simulink model "AutoPID_FOC_Model_Voltage"  (R2022b)
settings: Solver=ode15s  StartTime=0.0  StopTime=5  MaxStep=1e-5  RelTol=1e-4
undefined symbols (not defined in the file): J, kc, p, PID_angle_limit, PID_vel_D, PID_vel_I, PID_vel_limit, PID_vel_output_ramp, PID_vel_P, step_final, Ts_control
libraries: fl_lib x6, nesl_utility x6, slpidlib x2, mcbcontrolslib x2, ee_lib x1
settings Model: Creator=ngryaznov  LastModifiedBy=ngryaznov
settings DataIOCC: SaveOutput=off  SignalLogging=off  SaveTime=off

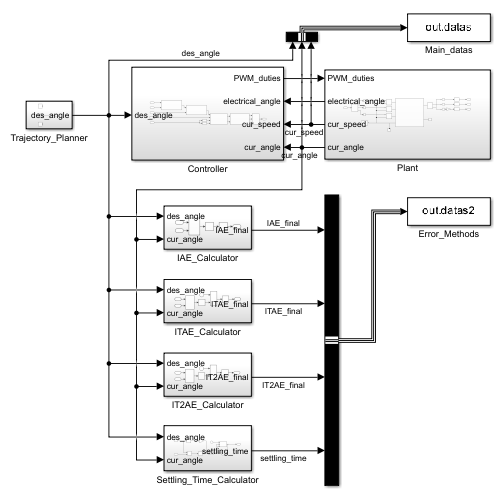
[thumbnail: Simulink's stored preview of the top-level diagram]
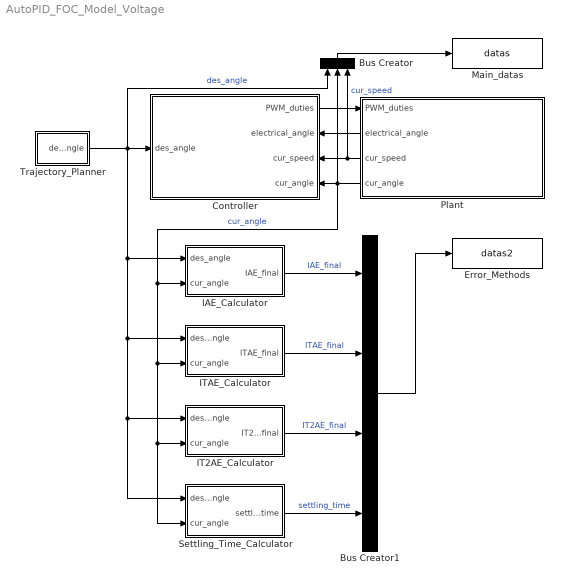
== system AutoPID_FOC_Model_Voltage ==
  Bus Creator : BusCreator  Inputs=3
  Bus Creator1 : BusCreator  Inputs=4
  Controller : Subsystem
      settings: PortSchema="{\"entries\":[{\"content\":{\"sides\":[{\"content\":{\"connectorIds\":[\"In1\"]},\"type\":\"ConnectorPlacement.EquallySpacedRectSide\",\"uuid\":\"0423d24d-9521-4525-a0e4-a3e2e668f0ac\"},{\"content\":{\"connectorIds\":[\"Out1\",\"In2\",\"In3\",\"In4\"],\"side\":\"RIGHT\"},\"type\":\"ConnectorPlacement.EquallySpacedRectSide\",\"uuid\":\"47c71c52-a907-4714-8b3c-a2837c55c5aa\"},{\"content\":{\"connectorIds\":[],\"side\":\"TOP\"},\"type\":\"ConnectorPlacement.EquallySpacedRectSide\",\"uuid\":\"3c8a956e-8d48-45c8-90f9-0152c5abea5b\"}]},\"type\":\"ConnectorPlacement.EquallySpacedConnector\",\"uuid\":\"215a3bc6-e4d0-4bbf-a22d-a4a170c152a2\"}],\"packageUris\":[\"http://schema.mathworks.com/mf0/Connector/R2020b\"],\"version\":\"1.0\"}"
  Error_Methods : ToWorkspace  VariableName=datas2  SaveFormat=Timeseries  SampleTime=-1
      settings: Decimation=2
  IAE_Calculator : Subsystem
  IT2AE_Calculator : Subsystem
  ITAE_Calculator : Subsystem
  Main_datas : ToWorkspace  VariableName=datas  SaveFormat=Timeseries  SampleTime=-1
      settings: Decimation=2
  Plant : Subsystem
      settings: PortSchema="{\"entries\":[{\"content\":{\"sides\":[{\"content\":{\"connectorIds\":[\"In1\",\"Out1\",\"Out2\",\"Out3\"]},\"type\":\"ConnectorPlacement.EquallySpacedRectSide\",\"uuid\":\"e046dd69-40e9-406a-bd4f-9d09bb11ef1b\"},{\"content\":{\"connectorIds\":[],\"side\":\"RIGHT\"},\"type\":\"ConnectorPlacement.EquallySpacedRectSide\",\"uuid\":\"7e51beb7-44f5-4f8e-b575-c3917b5b8c79\"},{\"content\":{\"connectorIds\":[],\"side\":\"TOP\"},\"type\":\"ConnectorPlacement.EquallySpacedRectSide\",\"uuid\":\"ce36b3ae-82b4-4f86-a013-a2335df0f3e3\"}]},\"type\":\"ConnectorPlacement.EquallySpacedConnector\",\"uuid\":\"95338947-5a02-4018-9bff-e920c50d3b4f\"}],\"packageUris\":[\"http://schema.mathworks.com/mf0/Connector/R2020b\"],\"version\":\"1.0\"}"
  Settling_Time_Calculator : Subsystem
  Trajectory_Planner : Subsystem
  wires:
  Trajectory_Planner/1(des_angle) -> ITAE_Calculator/1(des_angle), IT2AE_Calculator/1(des_angle), Settling_Time_Calculator/1(des_angle), IAE_Calculator/1(des_angle), Controller/1(des_angle), Bus Creator/1  "des_angle"
  Controller/1(PWM_duties) -> Plant/1(PWM_duties)
  Plant/1(electrical_angle) -> Controller/2(electrical_angle)
  Plant/2(cur_speed) -> Bus Creator/3, Controller/3(cur_speed)  "cur_speed"
  Plant/3(cur_angle) -> Bus Creator/2, Controller/4(cur_angle), IAE_Calculator/2(cur_angle), ITAE_Calculator/2(cur_angle), IT2AE_Calculator/2(cur_angle), Settling_Time_Calculator/2(cur_angle)  "cur_angle"
  Bus Creator/1 -> Main_datas/1
  IAE_Calculator/1(IAE_final) -> Bus Creator1/1  "IAE_final"
  ITAE_Calculator/1(ITAE_final) -> Bus Creator1/2  "ITAE_final"
  IT2AE_Calculator/1(IT2AE_final) -> Bus Creator1/3  "IT2AE_final"
  Settling_Time_Calculator/1(settling_time) -> Bus Creator1/4  "settling_time"
  Bus Creator1/1 -> Error_Methods/1

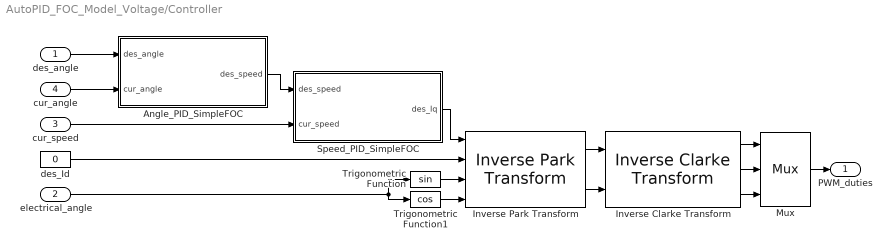
== system AutoPID_FOC_Model_Voltage/Controller ==
  des_angle : Inport
  electrical_angle : Inport  Port=2
  cur_speed : Inport  Port=3
  cur_angle : Inport  Port=4
  Angle_PID_SimpleFOC : Subsystem
  Inverse Clarke Transform : mcbcontrolslib/Inverse Clarke Transform
      settings: LibrarySourceBlock=mcblib/Controls/Math Transforms/Inverse Clarke Transform
  Inverse Park Transform : mcbcontrolslib/Inverse Park Transform  AxisAlignment=Q-axis
      settings: LibrarySourceBlock=mcblib/Controls/Math Transforms/Inverse Park Transform
  Mux : Mux  Inputs=3
      settings: DisplayOption=signals
  Speed_PID_SimpleFOC : Subsystem
  Trigonometric Function : Trigonometry
  Trigonometric Function1 : Trigonometry  Operator=cos
  des_Id : Constant  Value=0
  PWM_duties : Outport
  wires:
  des_angle/1 -> Angle_PID_SimpleFOC/1(des_angle)
  cur_angle/1 -> Angle_PID_SimpleFOC/2(cur_angle)
  des_Id/1 -> Inverse Park Transform/2
  electrical_angle/1 -> Trigonometric Function1/1, Trigonometric Function/1
  Trigonometric Function/1 -> Inverse Park Transform/3
  Trigonometric Function1/1 -> Inverse Park Transform/4
  Inverse Park Transform/2 -> Inverse Clarke Transform/2
  Mux/1 -> PWM_duties/1
  Inverse Clarke Transform/1 -> Mux/1
  Inverse Clarke Transform/3 -> Mux/3
  Inverse Clarke Transform/2 -> Mux/2
  Angle_PID_SimpleFOC/1(des_speed) -> Speed_PID_SimpleFOC/1(des_speed)
  cur_speed/1 -> Speed_PID_SimpleFOC/2(cur_speed)
  Inverse Park Transform/1 -> Inverse Clarke Transform/1
  Speed_PID_SimpleFOC/1(des_Iq) -> Inverse Park Transform/1

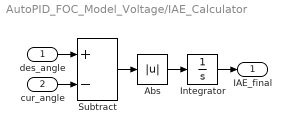
== system AutoPID_FOC_Model_Voltage/IAE_Calculator ==
  des_angle : Inport
  cur_angle : Inport  Port=2
  Abs : Abs  SaturateOnIntegerOverflow=off
  Integrator : Integrator
  Subtract : Sum  Inputs=+-
  IAE_final : Outport
  wires:
  Subtract/1 -> Abs/1
  des_angle/1 -> Subtract/1
  cur_angle/1 -> Subtract/2
  Integrator/1 -> IAE_final/1
  Abs/1 -> Integrator/1

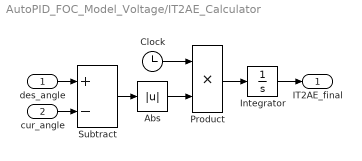
== system AutoPID_FOC_Model_Voltage/IT2AE_Calculator ==
  des_angle : Inport
  cur_angle : Inport  Port=2
  Abs : Abs  SaturateOnIntegerOverflow=off
  Clock : Clock
  Integrator : Integrator
  Product : Product
  Subtract : Sum  Inputs=+-
  IT2AE_final : Outport
  wires:
  des_angle/1 -> Subtract/1
  cur_angle/1 -> Subtract/2
  Subtract/1 -> Abs/1
  Abs/1 -> Product/2
  Clock/1 -> Product/1
  Integrator/1 -> IT2AE_final/1
  Product/1 -> Integrator/1

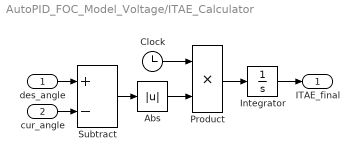
== system AutoPID_FOC_Model_Voltage/ITAE_Calculator ==
  des_angle : Inport
  cur_angle : Inport  Port=2
  Abs : Abs  SaturateOnIntegerOverflow=off
  Clock : Clock
  Integrator : Integrator
  Product : Product
  Subtract : Sum  Inputs=+-
  ITAE_final : Outport
  wires:
  Integrator/1 -> ITAE_final/1
  cur_angle/1 -> Subtract/2
  Subtract/1 -> Abs/1
  des_angle/1 -> Subtract/1
  Abs/1 -> Product/2
  Product/1 -> Integrator/1
  Clock/1 -> Product/1

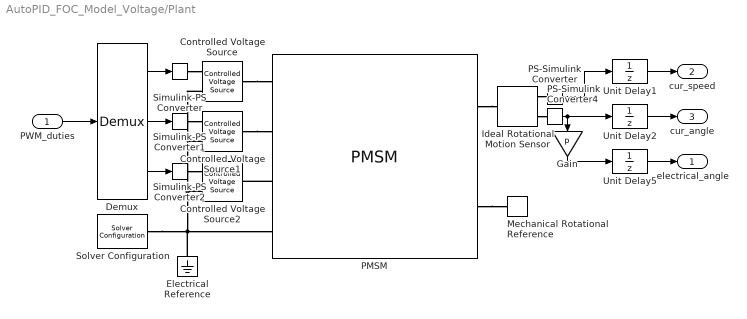
== system AutoPID_FOC_Model_Voltage/Plant ==
  PWM_duties : Inport
  Controlled Voltage Source : fl_lib/Electrical/Electrical Sources/Controlled Voltage Source
  Controlled Voltage Source1 : fl_lib/Electrical/Electrical Sources/Controlled Voltage Source
  Controlled Voltage Source2 : fl_lib/Electrical/Electrical Sources/Controlled Voltage Source
  Demux : Demux  Outputs=3
      settings: DisplayOption=none
  Electrical Reference : fl_lib/Electrical/Electrical Elements/Electrical Reference
  Gain : Gain  Gain=p
  Ideal Rotational Motion Sensor : fl_lib/Mechanical/Mechanical Sensors/Ideal Rotational Motion Sensor  reference=foundation.enum.MeasurementReference.absolute  acceleration_port=false  velocity_port=true  position_port=true  wrap_angle=false  offset=0 rad
      settings: InternalSimscapePortConfiguration="{\"Bottom\":[],\"Left\":[{\"id\":\"R\",\"label\":\"R\",\"type\":\"foundation.mechanical.rotational.rotational\"}],\"Right\":[{\"id\":\"W\",\"label\":\"W\",\"type\":\"output\"},{\"id\":\"A\",\"label\":\"A\",\"type\":\"output\"}],\"Top\":[]}"
  Mechanical Rotational Reference : fl_lib/Mechanical/Rotational Elements/Mechanical Rotational Reference
  PMSM : ee_lib/Electromechanical/Permanent Magnet/PMSM  port_option=ee.enum.threePhasePort.expanded  winding_type=ee.enum.statorconnection.wye  machine_param=ee.enum.pmsm.parameterization.constant  nPolePairs=p  pmflux_param=ee.enum.pmflux.fluxlinkage  pm_flux_linkage=lambda_pm Wb  torque_constant=0.18 N*m/A  back_emf_constant=0.18 V*s/rad  stator_param=ee.enum.statorparam.LdLqL0  Ld=Ld H  Lq=Lq H  idVec=[-200, 0, 200] A  iqVec=[-200, 0, 200] A  LdMatrix=0.0002 * ones(3, 3) H  LqMatrix=0.0002 * ones(3, 3) H  PmMatrix=0.1 * ones(3, 3) Wb  ktMatrix=0.18 * ones(3, 3) N*m/A  keMatrix=0.18 * ones(3, 3) V*s/rad  L0=Ld H  Ls=0.0002 H  Lm=-0.00002 H  Ms=0.00002 H  Rs=Rs Ohm  zero_sequence=ee.enum.park.zerosequence.include  axes_param=ee.enum.rotorangle.daxis  loss_param=ee.enum.ironloss.none  losses_oc=[0, 0, 0] W  losses_sc=[0, 0, 0] W  f_losses=60 Hz  Isc_losses=95 A  J=J kg*m^2  lam=B N*m*s/rad  i_d_specify=off  i_d_priority=None  i_d=0 A  i_d_nominal_specify=off  i_d_nominal_unit=A  i_d_nominal_value=1  i_q_specify=off  i_q_priority=None  i_q=0 A  i_q_nominal_specify=off  i_q_nominal_unit=A  i_q_nominal_value=1  torque_specify=off  torque_priority=None  torque=0 N*m  torque_nominal_specify=off  torque_nominal_unit=N*m  torque_nominal_value=1  angular_velocity_specify=off  angular_velocity_priority=High  angular_velocity=0 rpm  angular_velocity_nominal_specify=off  angular_velocity_nominal_unit=rpm  angular_velocity_nominal_value=1  angular_position_specify=off  angular_position_priority=High  angular_position=0 deg  angular_position_nominal_specify=off  angular_position_nominal_unit=deg  angular_position_nominal_value=1  alpha=3.93e-3 1/K  alpha_flux=-0.001 1/K  Tmeas=298.15 K  stator_thermal_mass=100 J/K  rotor_thermal_mass=200 J/K  Rm_percent_rotor=90  Rd_percent_rotor=30  temperatureA_specify=off  temperatureA_priority=High  temperatureA=25 degC  temperatureA_nominal_specify=off  temperatureA_nominal_unit=degC  temperatureA_nominal_value=1  temperatureB_specify=off  temperatureB_priority=High  temperatureB=25 degC  temperatureB_nominal_specify=off  temperatureB_nominal_unit=degC  temperatureB_nominal_value=1  temperatureC_specify=off  temperatureC_priority=High  temperatureC=25 degC  temperatureC_nominal_specify=off  temperatureC_nominal_unit=degC  temperatureC_nominal_value=1  temperatureR_specify=off  temperatureR_priority=High  temperatureR=25 degC  temperatureR_nominal_specify=off  temperatureR_nominal_unit=degC  temperatureR_nominal_value=1
      settings: InternalSimscapePortConfiguration="{\"Bottom\":[],\"Left\":[{\"id\":\"a\",\"label\":\"a\",\"type\":\"foundation.electrical.electrical\"},{\"id\":\"b\",\"label\":\"b\",\"type\":\"foundation.electrical.electrical\"},{\"id\":\"c\",\"label\":\"c\",\"type\":\"foundation.electrical.electrical\"},{\"id\":\"n\",\"label\":\"n\",\"type\":\"foundation.electrical.electrical\"}],\"Right\":[{\"id\":\"R\",\"label\":\"R\",\"type\":\"foundation.mechanical.rotational.rotational\"},{\"id\":\"C\",\"label\":\"C\",\"type\":\"foundation.mechanical.rotational.rotational\"}],\"Top\":[]}"
  PS-Simulink Converter : nesl_utility/PS-Simulink Converter  PhysicalDomain=network_engine_domain  SubClassName=ps_output  LeftPortType=input  RightPortType=output  PseudoPeriodic=off  Frequencies=[]  VectorFormat=inherit  Unit=inherit  AffineConversion=off
  PS-Simulink Converter4 : nesl_utility/PS-Simulink Converter  PhysicalDomain=network_engine_domain  SubClassName=ps_output  LeftPortType=input  RightPortType=output  PseudoPeriodic=off  Frequencies=[]  VectorFormat=inherit  Unit=inherit  AffineConversion=off
  Simulink-PS Converter : nesl_utility/Simulink-PS Converter  PhysicalDomain=network_engine_domain  SubClassName=ps_input  LeftPortType=input  RightPortType=output  PseudoPeriodic=off  Frequencies=[]  NoiseDistribution=none  NoiseParameters=[]  Unit=1  AffineConversion=off  FilteringAndDerivatives=provide  SimscapeFilterOrder=1  InputFilterTimeConstant=0.001  UdotUserProvided=0
  Simulink-PS Converter1 : nesl_utility/Simulink-PS Converter  PhysicalDomain=network_engine_domain  SubClassName=ps_input  LeftPortType=input  RightPortType=output  PseudoPeriodic=off  Frequencies=[]  NoiseDistribution=none  NoiseParameters=[]  Unit=1  AffineConversion=off  FilteringAndDerivatives=provide  SimscapeFilterOrder=1  InputFilterTimeConstant=0.001  UdotUserProvided=0
  Simulink-PS Converter2 : nesl_utility/Simulink-PS Converter  PhysicalDomain=network_engine_domain  SubClassName=ps_input  LeftPortType=input  RightPortType=output  PseudoPeriodic=off  Frequencies=[]  NoiseDistribution=none  NoiseParameters=[]  Unit=1  AffineConversion=off  FilteringAndDerivatives=provide  SimscapeFilterOrder=1  InputFilterTimeConstant=0.001  UdotUserProvided=0
  Solver Configuration : nesl_utility/Solver Configuration  PhysicalDomain=network_engine_domain  SubClassName=solver  LeftPortType=input  RightPortType=generic  Tones=[]  Harmonics=[]  SimulateNoise=off  Profile=off  UseLocalSampling=off  EnableSwitchedLinearOptims=on  FrequencyDomain=off  UseCCode=off  RelTol=0.001  AbsTol=0.001  MinStep=1e-09  ToWorkspace=off  RevertToSquareIcSolve=off  NumHomotopyIterations=100  PhasorMode=off  PhasorModeNumHarmonics=1  ConsistencySolver=NEWTON_XTOL_AFTER_FTOL  IndexReductionMethod=DerivativeReplacement  DoDC=off  ResidualTolerance=1e-09  ConsistencyTolSource=GLOBAL  ConsistencyAbsTol=0.001  ConsistencyRelTol=0.001  ConsistencyTolFactor=0.001  UseLocalSolver=on  LocalSolverChoice=NE_BACKWARD_EULER_ADVANCER  ResolveIndetEquations=on  FunctionEvalNumThread=1  LocalSolverSampleTime=0.001  DoFixedCost=on  MaxNonlinIter=3  MaxModeIter=2  ComputeImpulses=off  ImpulseIterations=2  LinearAlgebra=auto  LinearAlgebraNumThread=0  EquationFormulation=NE_TIME_EF  DelaysMemoryBudget=1024  AutomaticFiltering=on  FilteringTimeConstant=0.001  PartitionStorageMethod=AS_NEEDED  PartitionMemoryBudget=1024  PartitionMethod=ROBUST
  Unit Delay1 : UnitDelay  SampleTime=Ts_control  HasFrameUpgradeWarning=on
  Unit Delay2 : UnitDelay  SampleTime=Ts_control  HasFrameUpgradeWarning=on
  Unit Delay5 : UnitDelay  SampleTime=Ts_control  HasFrameUpgradeWarning=on
  electrical_angle : Outport
  cur_speed : Outport  Port=2
  cur_angle : Outport  Port=3
  wires:
  PS-Simulink Converter/1 -> Unit Delay1/1
  PS-Simulink Converter4/1 -> Unit Delay2/1, Gain/1
  PWM_duties/1 -> Demux/1
  Gain/1 -> Unit Delay5/1
  Demux/1 -> Simulink-PS Converter/1
  Demux/2 -> Simulink-PS Converter1/1
  Demux/3 -> Simulink-PS Converter2/1
  Unit Delay1/1 -> cur_speed/1
  Unit Delay2/1 -> cur_angle/1
  Unit Delay5/1 -> electrical_angle/1
  connections:
  Simulink-PS Converter/RConn1 -- Controlled Voltage Source/RConn1
  Simulink-PS Converter1/RConn1 -- Controlled Voltage Source1/RConn1
  Simulink-PS Converter2/RConn1 -- Controlled Voltage Source2/RConn1
  PMSM/LConn3 -- Controlled Voltage Source2/LConn1
  Controlled Voltage Source/LConn1 -- PMSM/LConn1
  Controlled Voltage Source1/LConn1 -- PMSM/LConn2
  Electrical Reference/LConn1 -- Solver Configuration/RConn1 -- PMSM/LConn4 -- Controlled Voltage Source/RConn2 -- Controlled Voltage Source1/RConn2 -- Controlled Voltage Source2/RConn2
  PMSM/RConn1 -- Ideal Rotational Motion Sensor/LConn1
  Ideal Rotational Motion Sensor/RConn1 -- PS-Simulink Converter/LConn1
  PMSM/RConn2 -- Mechanical Rotational Reference/LConn1
  Ideal Rotational Motion Sensor/RConn2 -- PS-Simulink Converter4/LConn1

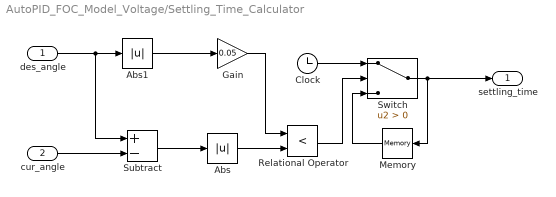
== system AutoPID_FOC_Model_Voltage/Settling_Time_Calculator ==
  des_angle : Inport
  cur_angle : Inport  Port=2
  Abs : Abs  SaturateOnIntegerOverflow=off
  Abs1 : Abs  SaturateOnIntegerOverflow=off
  Clock : Clock
  Gain : Gain  Gain=0.05
  Memory : Memory
  Relational Operator : RelationalOperator  Operator=<  OutDataTypeStr=boolean  RndMeth=Simplest  InputSameDT=off
  Subtract : Sum  Inputs=+-
  Switch : Switch  Criteria=u2 > Threshold  SaturateOnIntegerOverflow=off  InputSameDT=off
  settling_time : Outport
  wires:
  des_angle/1 -> Subtract/1, Abs1/1
  cur_angle/1 -> Subtract/2
  Subtract/1 -> Abs/1
  Abs1/1 -> Gain/1
  Gain/1 -> Relational Operator/1
  Abs/1 -> Relational Operator/2
  Clock/1 -> Switch/1
  Relational Operator/1 -> Switch/2
  Switch/1 -> settling_time/1, Memory/1
  Memory/1 -> Switch/3

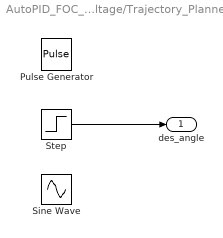
== system AutoPID_FOC_Model_Voltage/Trajectory_Planner ==
  Pulse Generator : DiscretePulseGenerator  PulseType=Time based  Period=5  PulseWidth=50
  Sine Wave : Sin  Frequency=2*pi*0.1  SampleTime=0
  Step : Step  Time=0.01  After=step_final  SampleTime=Ts_control
  des_angle : Outport
  wires:
  Step/1 -> des_angle/1

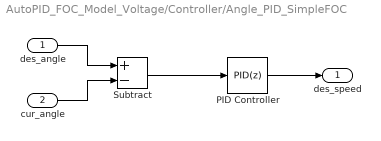
== system AutoPID_FOC_Model_Voltage/Controller/Angle_PID_SimpleFOC ==
  des_angle : Inport
  cur_angle : Inport  Port=2
  PID Controller : slpidlib/PID Controller  Controller=PID  Form=Parallel  TimeDomain=Discrete-time  UseExternalTs=off  SampleTime=Ts_control  IntegratorMethod=Trapezoidal  FilterMethod=Trapezoidal  ControllerParametersSource=internal  P=PID_vel_P  I=PID_vel_I  UseKiTs=off  D=PID_vel_D  N=100  UseFilter=on  TunerSelectOption=Transfer Function Based (PID Tuner App)  InitialConditionSource=internal  InitialConditionForIntegrator=0  InitialConditionForFilter=0  DifferentiatorICPrevScaledInput=0  ExternalReset=none  TrackingMode=off  Kt=1  LimitOutput=on  SatLimitsSource=internal  UpperSaturationLimit=PID_angle_limit  LowerSaturationLimit=-PID_angle_limit  LinearizeAsGain=off  AntiWindupMode=back-calculation  Kb=kc  LimitIntegrator=off  UpperIntegratorSaturationLimit=inf  LowerIntegratorSaturationLimit=-inf  POutMin=[]  POutMax=[]  IOutMin=[]  IOutMax=[]  DOutMin=[]  DOutMax=[]  NOutMin=[]  NOutMax=[]  SumOutMin=[]  SumOutMax=[]  SaturationOutMin=[]  SaturationOutMax=[]  PParamMin=[]  PParamMax=[]  IParamMin=[]  IParamMax=[]  DParamMin=[]  DParamMax=[]  NParamMin=[]  NParamMax=[]  KbParamMin=[]  KbParamMax=[]  KtParamMin=[]  KtParamMax=[]  KbOutMin=[]  KbOutMax=[]  KtOutMin=[]  KtOutMax=[]  IntegratorOutMin=[]  IntegratorOutMax=[]  FilterOutMin=[]  FilterOutMax=[]  SumI1OutMin=[]  SumI1OutMax=[]  SumI2OutMin=[]  SumI2OutMax=[]  SumI3OutMin=[]  SumI3OutMax=[]  SumI4OutMin=[]  SumI4OutMax=[]  SumDOutMin=[]  SumDOutMax=[]  DifferentiatorOutMin=[]  DifferentiatorOutMax=[]  FilterDiffOutCoefMin=[]  FilterDiffOutCoefMax=[]  ReciprocalOutMin=[]  ReciprocalOutMax=[]  SumDenOutMin=[]  SumDenOutMax=[]  SumNumOutMin=[]  SumNumOutMax=[]  DivideOutMin=[]  DivideOutMax=[]  UdiffTsProdOutMin=[]  UdiffTsProdOutMax=[]  NTsProdOutMin=[]  NTsProdOutMax=[]  UintegralTsProdOutMin=[]  UintegralTsProdOutMax=[]  UngainTsProdOutMin=[]  UngainTsProdOutMax=[]  ClampingZeroOutDataTypeStr=Inherit: Inherit via back propagation  ClampingZeroOutMin=[]  ClampingZeroOutMax=[]  FilterDenConstantOutDataTypeStr=Inherit: Inherit via back propagation  FilterDenConstantOutMin=[]  FilterDenConstantOutMax=[]  PCopyOutDataTypeStr=Inherit: Inherit via back propagation  PCopyOutMin=[]  PCopyOutMax=[]  NCopyOutDataTypeStr=Inherit: Inherit via back propagation  NCopyOutMin=[]  NCopyOutMax=[]  IntegratorContinuousStateAttributes=''  IntegratorStateMustResolveToSignalObject=off  IntegratorRTWStateStorageClass=Auto  FilterContinuousStateAttributes=''  FilterStateMustResolveToSignalObject=off  FilterRTWStateStorageClass=Auto  ParallelPVariant=InternalParameters  IdealPVariant=Disabled  IVariant=InternalParameters  DVariant=InternalParameters  IntegratorVariant=Discrete  SatVariant=Enabled  AWVariant=BackCalculation  PCopyVariant=Disabled  TRVariant=Disabled  FdbkBlocksVariant=Feedback  IdealPFdbkVariant=Passthrough  SatFdbkVariant=Enabled  DerivativeFilterVariant=TrapezoidalFilter  NVariant=InternalParameters  NCopyVariant=InternalParameters  FilterICVariant=InternalICsFilter  IntegratorICVariant=InternalICs  ExternalResetVariant=Disabled  TRSumVariant=Passthrough  SumFdbkVariant=Enabled  SumVariant=Sum_PID  TsampFilterVariant=InternalTs  TsampNgainVariant=Passthrough  TsampIntegralVariant=Passthrough  ExternalSaturationOutDataTypeStr=Inherit: Same as second input
  Subtract : Sum  Inputs=+-
  des_speed : Outport
  wires:
  des_angle/1 -> Subtract/1
  cur_angle/1 -> Subtract/2
  Subtract/1 -> PID Controller/1
  PID Controller/1 -> des_speed/1

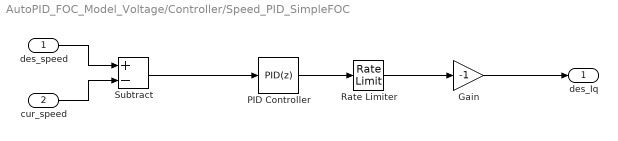
== system AutoPID_FOC_Model_Voltage/Controller/Speed_PID_SimpleFOC ==
  des_speed : Inport
  cur_speed : Inport  Port=2
  Gain : Gain  Gain=-1
  PID Controller : slpidlib/PID Controller  Controller=PID  Form=Parallel  TimeDomain=Discrete-time  UseExternalTs=off  SampleTime=Ts_control  IntegratorMethod=Trapezoidal  FilterMethod=Trapezoidal  ControllerParametersSource=internal  P=PID_vel_P  I=PID_vel_I  UseKiTs=off  D=PID_vel_D  N=100  UseFilter=on  TunerSelectOption=Transfer Function Based (PID Tuner App)  InitialConditionSource=internal  InitialConditionForIntegrator=0  InitialConditionForFilter=0  DifferentiatorICPrevScaledInput=0  ExternalReset=none  TrackingMode=off  Kt=1  LimitOutput=on  SatLimitsSource=internal  UpperSaturationLimit=PID_vel_limit  LowerSaturationLimit=-PID_vel_limit  LinearizeAsGain=off  AntiWindupMode=back-calculation  Kb=kc  LimitIntegrator=off  UpperIntegratorSaturationLimit=inf  LowerIntegratorSaturationLimit=-inf  POutMin=[]  POutMax=[]  IOutMin=[]  IOutMax=[]  DOutMin=[]  DOutMax=[]  NOutMin=[]  NOutMax=[]  SumOutMin=[]  SumOutMax=[]  SaturationOutMin=[]  SaturationOutMax=[]  PParamMin=[]  PParamMax=[]  IParamMin=[]  IParamMax=[]  DParamMin=[]  DParamMax=[]  NParamMin=[]  NParamMax=[]  KbParamMin=[]  KbParamMax=[]  KtParamMin=[]  KtParamMax=[]  KbOutMin=[]  KbOutMax=[]  KtOutMin=[]  KtOutMax=[]  IntegratorOutMin=[]  IntegratorOutMax=[]  FilterOutMin=[]  FilterOutMax=[]  SumI1OutMin=[]  SumI1OutMax=[]  SumI2OutMin=[]  SumI2OutMax=[]  SumI3OutMin=[]  SumI3OutMax=[]  SumI4OutMin=[]  SumI4OutMax=[]  SumDOutMin=[]  SumDOutMax=[]  DifferentiatorOutMin=[]  DifferentiatorOutMax=[]  FilterDiffOutCoefMin=[]  FilterDiffOutCoefMax=[]  ReciprocalOutMin=[]  ReciprocalOutMax=[]  SumDenOutMin=[]  SumDenOutMax=[]  SumNumOutMin=[]  SumNumOutMax=[]  DivideOutMin=[]  DivideOutMax=[]  UdiffTsProdOutMin=[]  UdiffTsProdOutMax=[]  NTsProdOutMin=[]  NTsProdOutMax=[]  UintegralTsProdOutMin=[]  UintegralTsProdOutMax=[]  UngainTsProdOutMin=[]  UngainTsProdOutMax=[]  ClampingZeroOutDataTypeStr=Inherit: Inherit via back propagation  ClampingZeroOutMin=[]  ClampingZeroOutMax=[]  FilterDenConstantOutDataTypeStr=Inherit: Inherit via back propagation  FilterDenConstantOutMin=[]  FilterDenConstantOutMax=[]  PCopyOutDataTypeStr=Inherit: Inherit via back propagation  PCopyOutMin=[]  PCopyOutMax=[]  NCopyOutDataTypeStr=Inherit: Inherit via back propagation  NCopyOutMin=[]  NCopyOutMax=[]  IntegratorContinuousStateAttributes=''  IntegratorStateMustResolveToSignalObject=off  IntegratorRTWStateStorageClass=Auto  FilterContinuousStateAttributes=''  FilterStateMustResolveToSignalObject=off  FilterRTWStateStorageClass=Auto  ParallelPVariant=InternalParameters  IdealPVariant=Disabled  IVariant=InternalParameters  DVariant=InternalParameters  IntegratorVariant=Discrete  SatVariant=Enabled  AWVariant=BackCalculation  PCopyVariant=Disabled  TRVariant=Disabled  FdbkBlocksVariant=Feedback  IdealPFdbkVariant=Passthrough  SatFdbkVariant=Enabled  DerivativeFilterVariant=TrapezoidalFilter  NVariant=InternalParameters  NCopyVariant=InternalParameters  FilterICVariant=InternalICsFilter  IntegratorICVariant=InternalICs  ExternalResetVariant=Disabled  TRSumVariant=Passthrough  SumFdbkVariant=Enabled  SumVariant=Sum_PID  TsampFilterVariant=InternalTs  TsampNgainVariant=Passthrough  TsampIntegralVariant=Passthrough  ExternalSaturationOutDataTypeStr=Inherit: Same as second input
  Rate Limiter : RateLimiter  RisingSlewLimit=PID_vel_output_ramp  FallingSlewLimit=-PID_vel_output_ramp  SampleTimeMode=inherited
  Subtract : Sum  Inputs=+-
  des_Iq : Outport
  wires:
  des_speed/1 -> Subtract/1
  cur_speed/1 -> Subtract/2
  Subtract/1 -> PID Controller/1
  PID Controller/1 -> Rate Limiter/1
  Rate Limiter/1 -> Gain/1
  Gain/1 -> des_Iq/1
